simulink model "ex1dof"  (R2026a)
settings: Solver=VariableStepAuto
InitFcn:
  | airframe.m = 0.8;
  | 
  | w_m = 30.5;
  | w_washout = 50;
  | 
  | tau_m = 1/w_m;
  | tau_washout = 1/w_washout;
  | 
  | g = 9.81;
settings Model: Creator=devinbellll  LastModifiedBy=devinbellll

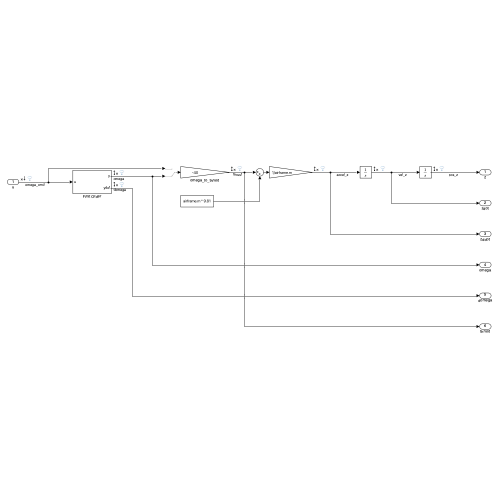
[thumbnail: Simulink's stored preview of the top-level diagram]
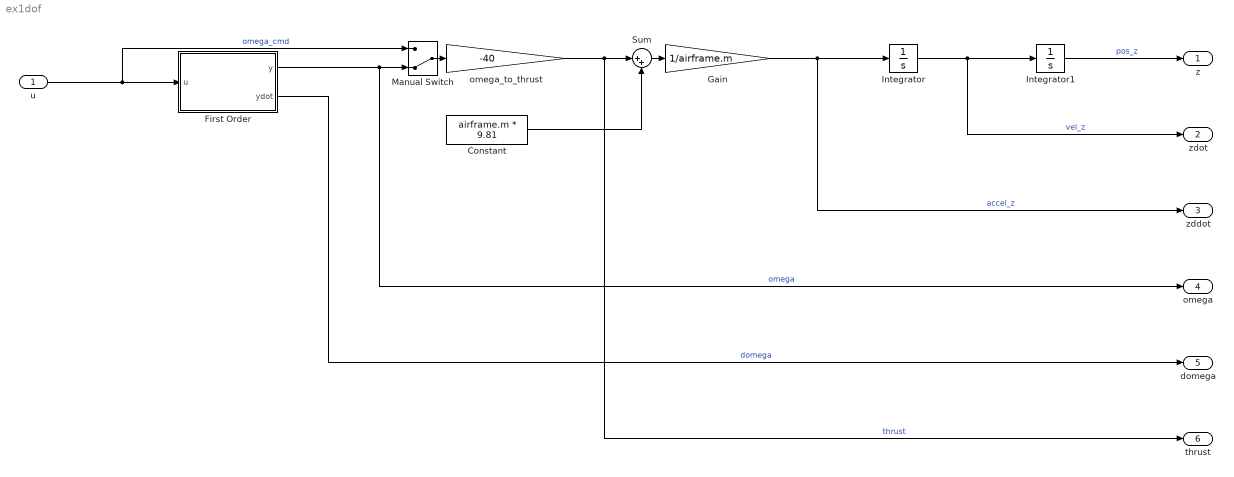
== system ex1dof ==
  u : Inport
  Constant : Constant  Value=airframe.m * 9.81
  First Order : Subsystem
  Gain : Gain  Gain=1/airframe.m
  Integrator : Integrator  ContinuousStateAttributes='zdot'
  Integrator1 : Integrator  ContinuousStateAttributes='z'
  Manual Switch : ManualSwitch  CurrentSetting=0
  Sum : Sum  Inputs=|++
  omega_to_thrust : Gain  Gain=-40
  z : Outport
  zdot : Outport  Port=2
  zddot : Outport  Port=3
  omega : Outport  Port=4
  domega : Outport  Port=5
  thrust : Outport  Port=6
  wires:
  Integrator/1 -> zdot/1, Integrator1/1  "vel_z"
  Integrator1/1 -> z/1  "pos_z"
  Gain/1 -> zddot/1, Integrator/1  "accel_z"
  omega_to_thrust/1 -> Sum/1, thrust/1  "thrust"
  First Order/1(y) -> Manual Switch/2, omega/1  "omega"
  First Order/2(ydot) -> domega/1  "domega"
  u/1 -> Manual Switch/1, First Order/1(u)  "omega_cmd"
  Sum/1 -> Gain/1
  Constant/1 -> Sum/2
  Manual Switch/1 -> omega_to_thrust/1

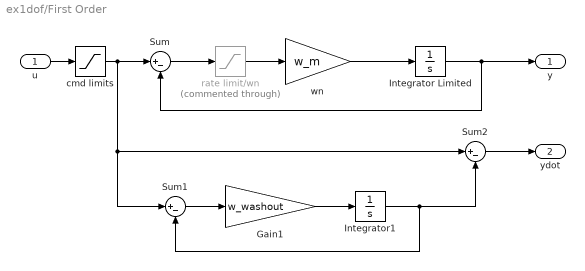
== system ex1dof/First Order ==
  u : Inport
  Gain1 : Gain  Gain=w_washout
  Integrator Limited : Integrator  InitialCondition=(airframe.m * 9.81) / 40  LimitOutput=on  UpperSaturationLimit=1  LowerSaturationLimit=0  ContinuousStateAttributes='omega'
  Integrator1 : Integrator  ContinuousStateAttributes='omega_dot'
  Sum : Sum  Inputs=|+-
  Sum1 : Sum  Inputs=|+-
  Sum2 : Sum  Inputs=|+-
  cmd limits : Saturate  UpperLimit=1  LowerLimit=0
  rate limit/wn : Saturate  Commented=through
  wn : Gain  Gain=w_m
  y : Outport
  ydot : Outport  Port=2
  wires:
  cmd limits/1 -> Sum/1, Sum1/1, Sum2/1
  Sum/1 -> rate limit/wn/1
  wn/1 -> Integrator Limited/1
  Integrator Limited/1 -> Sum/2, y/1
  rate limit/wn/1 -> wn/1
  Sum2/1 -> ydot/1
  Gain1/1 -> Integrator1/1
  Sum1/1 -> Gain1/1
  u/1 -> cmd limits/1
  Integrator1/1 -> Sum2/2, Sum1/2
